simulink model "RC_circuit"  (R2020a)
settings: Solver=VariableStepAuto  StartTime=0.0  StopTime=10.0  MaxStep=0.001  RelTol=1e-3
values from neighbouring files (symbols this model uses):
  C = 10 * 10^(-6)    (= 1e-05)    [DefaultValues.m]
  R = 10    [DefaultValues.m]
settings Model: Creator=DELL  LastModifiedBy=DELL

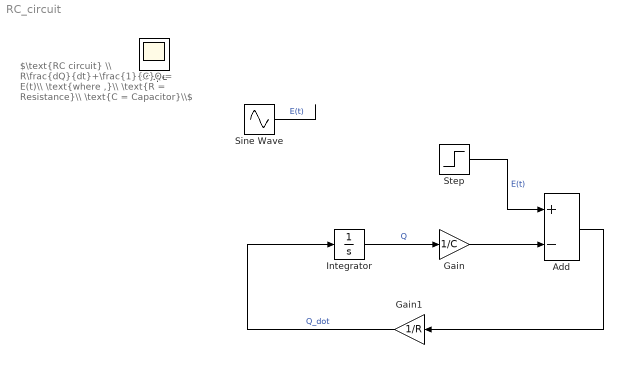
== system RC_circuit ==
  note: $\text{RC circuit} \\ R\frac{dQ}{dt}+\frac{1}{C}Q = E(t)\\ \text{where ,}\\ \text{R = Resistance}\\ \text{C = Capacitor}\\$
  Add : Sum  Inputs=+-
  Gain : Gain  Gain=1/C
  Gain1 : Gain  Gain=1/R
  Integrator : Integrator  InitialCondition=0.01
  Sine Wave : Sin  Amplitude=10  Frequency=2*pi*50  SampleTime=0
  Step : Step  SampleTime=0
  Scope : Scope
  wires:
  Gain1/1 -> Integrator/1  "Q_dot"
  Integrator/1 -> Gain/1  "Q"
  Gain/1 -> Add/2
  Add/1 -> Gain1/1
  Step/1 -> Add/1  "E(t)"
  Sine Wave/1 -> ?  "E(t)"
